simulink library "INT_CoVeh_TrqLeadCoord"  (R2016b)
settings: Solver=VariableStepAuto  StartTime=0.0  StopTime=10.0  RelTol=1e-3
settings Model: Creator=Administrator  LastModifiedBy=Administrator

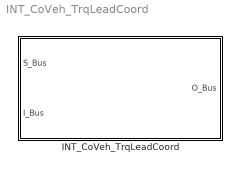
== system INT_CoVeh_TrqLeadCoord ==
  INT_CoVeh_TrqLeadCoord : Subsystem

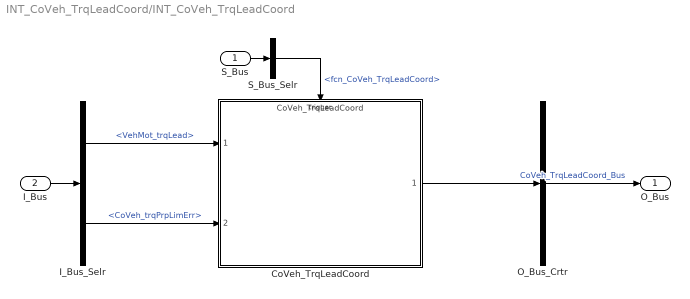
== system INT_CoVeh_TrqLeadCoord/INT_CoVeh_TrqLeadCoord ==
  S_Bus : Inport
  I_Bus : Inport  Port=2
  CoVeh_TrqLeadCoord : ModelReference  ModelNameDialog=CoVeh_TrqLeadCoord  SimulationMode=Normal  ModelReferenceVersion=1.4  TriggerPortName=function  TriggerPortTriggerType=function-call  TriggerPortStatesWhenEnabling=held
  I_Bus_Selr : BusSelector  OutputSignals=VehMot_trqLead,CoVeh_trqPrpLimErr
  O_Bus_Crtr : BusCreator  Inputs=1
  S_Bus_Selr : BusSelector  OutputSignals=fcn_CoVeh_TrqLeadCoord
  O_Bus : Outport
  wires:
  S_Bus_Selr/1 -> CoVeh_TrqLeadCoord/Trigger  "<fcn_CoVeh_TrqLeadCoord>"
  S_Bus/1 -> S_Bus_Selr/1
  I_Bus/1 -> I_Bus_Selr/1
  I_Bus_Selr/1 -> CoVeh_TrqLeadCoord/1  "<VehMot_trqLead>"
  I_Bus_Selr/2 -> CoVeh_TrqLeadCoord/2  "<CoVeh_trqPrpLimErr>"
  O_Bus_Crtr/1 -> O_Bus/1  "CoVeh_TrqLeadCoord_Bus"
  CoVeh_TrqLeadCoord/1 -> O_Bus_Crtr/1
